simulink model "kallman"  (R2018a)
settings: Solver=VariableStepAuto  StartTime=0.0  StopTime=2  FixedStep=h  RelTol=1e-3
values from neighbouring files (symbols this model uses):
  AKC = Ad-Kk*Cd    [initLinSysID.m]
  Kk = Kk'    [initLinSysID.m]
undefined symbols (not defined in the file or in its folder): Bd
settings Model: Creator=geert  LastModifiedBy=geert

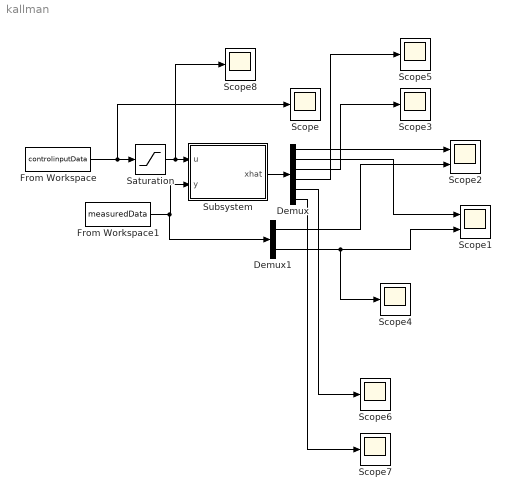
== system kallman ==
  Demux : Demux  Outputs=6
  Demux1 : Demux  Outputs=2
  From Workspace : FromWorkspace  VariableName=controlinputData
  From Workspace1 : FromWorkspace  VariableName=measuredData  SampleTime=0.001
  Saturation : Saturate  UpperLimit=1  LowerLimit=-1
  Scope{,3..8} (7 alike) : Scope
  Scope1 : Scope  NumInputPorts=2
  Scope2 : Scope  NumInputPorts=2
  Subsystem : Subsystem
  wires:
  From Workspace/1 -> Saturation/1, Scope/1
  From Workspace1/1 -> Subsystem/2(y), Demux1/1
  Subsystem/1(xhat) -> Demux/1
  Demux/1 -> Scope2/1
  Demux1/1 -> Scope2/2
  Demux/2 -> Scope1/1
  Demux1/2 -> Scope4/1, Scope1/2
  Demux/3 -> Scope3/1
  Demux/4 -> Scope5/1
  Demux/5 -> Scope6/1
  Demux/6 -> Scope7/1
  Saturation/1 -> Subsystem/1(u), Scope8/1

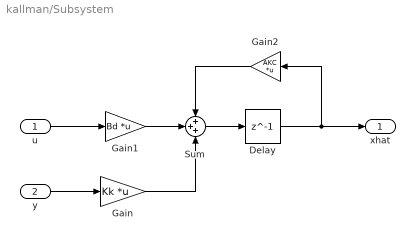
== system kallman/Subsystem ==
  u : Inport
  y : Inport  Port=2
  Delay : Delay  DelayLength=1
  Gain : Gain  Gain=Kk  Multiplication=Matrix(K*u)
  Gain1 : Gain  Gain=Bd  Multiplication=Matrix(K*u)
  Gain2 : Gain  Gain=AKC  Multiplication=Matrix(K*u)
  Sum : Sum  Inputs=+++
  xhat : Outport
  wires:
  Delay/1 -> Gain2/1, xhat/1
  y/1 -> Gain/1
  u/1 -> Gain1/1
  Sum/1 -> Delay/1
  Gain1/1 -> Sum/2
  Gain/1 -> Sum/3
  Gain2/1 -> Sum/1
